simulink model "Com_trafficl"  (R2020b)
settings: Solver=VariableStepAuto  StartTime=0.0  StopTime=10.0  RelTol=1e-3
settings Model: Creator=Taha  LastModifiedBy=Taha

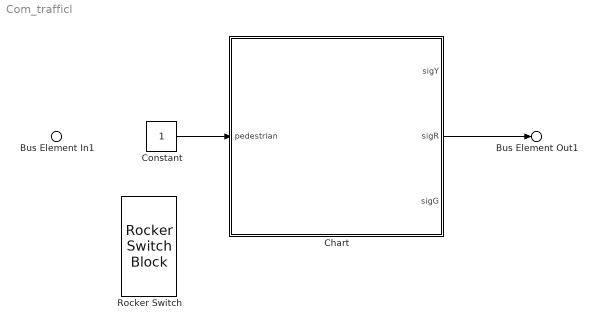
== system Com_trafficl ==
  Bus Element In1 : Inport  PortName=pedestrian
  Chart : Stateflow chart  TreatAsAtomicUnit=on
  Constant : Constant
  Rocker Switch : RockerSwitchBlock
      settings: Values={{'Off', 'On'}, [0 1]}
  Bus Element Out1 : Outport  PortName=sigR
  wires:
  Chart/2(sigR) -> Bus Element Out1/1
  Constant/1 -> Chart/1(pedestrian)

== stateflow chart Com_trafficl/Chart ==
  state GREEN
  state RED
  state PENDING
  state YELLOW
  GREEN -> GREEN [order 3] : [count < 60]{count = count + 1;}
  RED -> GREEN [order 1] : [count >= 60]{sigG = 1; count = 0}
  GREEN -> PENDING [order 1] : [pedestrian == 1 && count <60]{count = count +1;}
  GREEN -> YELLOW [order 2] : [pedestrian == 1 && count >= 60]{sigY = 1; count = 0;}
  (default) -> RED : {count =0;}
  RED -> RED [order 2] : {count = count + 1;}
  PENDING -> PENDING [order 2] : {count = count + 1;}
  YELLOW -> RED [order 1] : [count >= 5]{sigR = 1; count = 0;}
  PENDING -> YELLOW [order 1] : [count >= 60]{sigY = 1; count = 0;}
  YELLOW -> YELLOW [order 2] : {count = count + 1;}
  data: pedestrian input; sigY output; sigR output; sigG output; count local
